simulink model "Lab3_PID"  (R2021a)
settings: Solver=VariableStepAuto  StartTime=0.0  StopTime=10.0  RelTol=1e-3
settings Model: Creator=maria  LastModifiedBy=maria

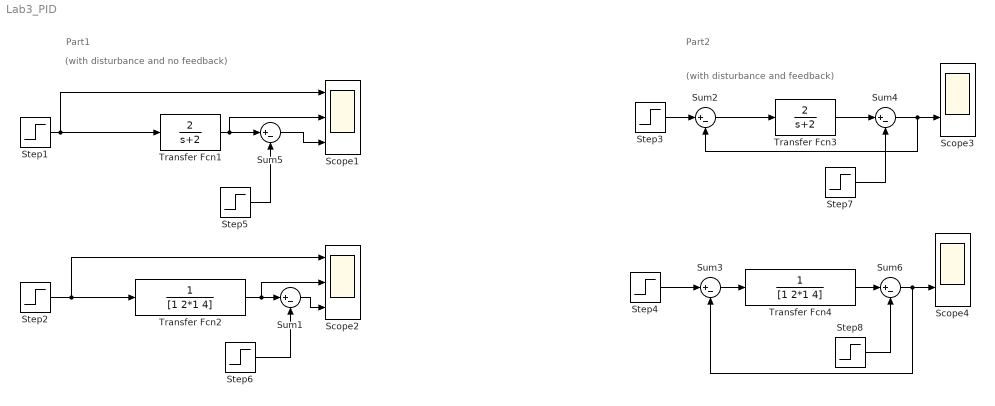
== system Lab3_PID ==
  note: (with disturbance and no feedback)
  note: Part1
  note: Part2
  note: (with disturbance and feedback)
  Scope1 : Scope  NumInputPorts=3
  Scope2 : Scope  NumInputPorts=3
  Scope3 : Scope  NumInputPorts=2
  Scope4 : Scope  NumInputPorts=2
  Step{1..2,5..7} (5 alike) : Step  SampleTime=0
  Step3 : Step  Time=3  After=0.7  SampleTime=0
  Step4 : Step  Time=3  After=0.7  SampleTime=0
  Step8 : Step  Time=5  After=0.3  SampleTime=0
  Sum{1..6} (6 alike) : Sum  Inputs=|+-
  Transfer Fcn1 : TransferFcn  Numerator=[2]  Denominator=[1 2]
  Transfer Fcn2 : TransferFcn  Denominator=[1 2*1 4]
  Transfer Fcn3 : TransferFcn  Numerator=[2]  Denominator=[1 2]
  Transfer Fcn4 : TransferFcn  Denominator=[1 2*1 4]
  wires:
  Step1/1 -> Scope1/1, Transfer Fcn1/1
  Step2/1 -> Scope2/1, Transfer Fcn2/1
  Sum2/1 -> Transfer Fcn3/1
  Step3/1 -> Sum2/1
  Step4/1 -> Sum3/1
  Sum3/1 -> Transfer Fcn4/1
  Transfer Fcn3/1 -> Sum4/1
  Sum4/1 -> Sum2/2, Scope3/2
  Transfer Fcn1/1 -> Scope1/2, Sum5/1
  Sum5/1 -> Scope1/3
  Step5/1 -> Sum5/2
  Sum1/1 -> Scope2/3
  Transfer Fcn2/1 -> Scope2/2, Sum1/1
  Step6/1 -> Sum1/2
  Step7/1 -> Sum4/2
  Transfer Fcn4/1 -> Sum6/1
  Sum6/1 -> Sum3/2, Scope4/2
  Step8/1 -> Sum6/2
